simulink model "new"  (R2023a)
settings: Solver=VariableStepAuto  StartTime=0.0  StopTime=4  RelTol=1e-3
values from neighbouring files (symbols this model uses):
  B = 0.0024    [I-PD_pole-placement.mat]    (also in PIV.mat; dobre_pid.mat; exam3.m; exam3_2.m)
  J_m = 0.005    [I-PD_pole-placement.mat]    (also in PIV.mat; dobre_pid.mat; exam3.m; exam3_2.m)
  k_i = 67.5    [I-PD_pole-placement.mat]    (also in PIV.mat = 2.36572; dobre_pid.mat = 0.0660293176822; exam3.m = 4.828; exam3_2.m)
  k_p = 7.6815    [I-PD_pole-placement.mat]    (also in PIV.mat = 5.79950289975; dobre_pid.mat = 8.78704740486; exam3.m = 8.2850041425; exam3_2.m)
  k_v = 0.16658    [PIV.mat]    (also in exam3.m = 0.239)
  M_n = 6.4    [I-PD_pole-placement.mat]    (also in PIV.mat; dobre_pid.mat; exam3.m; exam3_2.m)
  M_z0 = 0.033    [I-PD_pole-placement.mat]    (also in PIV.mat; dobre_pid.mat; exam3.m; exam3_2.m)
  Nel = 10000    [I-PD_pole-placement.mat]    (also in PIV.mat; dobre_pid.mat; exam3.m; exam3_2.m)
  T_n = 0.015    [I-PD_pole-placement.mat]    (also in PIV.mat; dobre_pid.mat; exam3.m; exam3_2.m)
  Tvz = 0.004    [I-PD_pole-placement.mat]    (also in PIV.mat; dobre_pid.mat; exam3.m; exam3_2.m)
undefined symbols (not defined in the file or in its folder): DiscIntNeverNeededParam
settings Model: Creator=laptop  LastModifiedBy=laptop

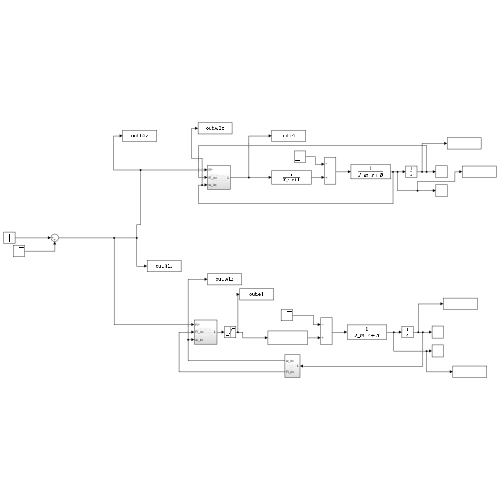
[thumbnail: Simulink's stored preview of the top-level diagram]
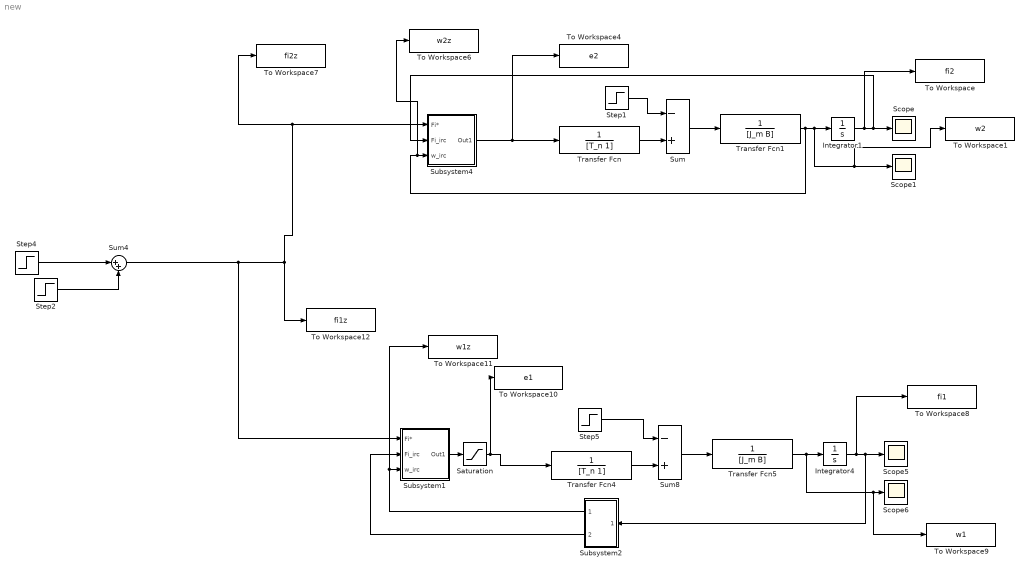
== system new ==
  Integrator1 : Integrator
  Integrator4 : Integrator
  Saturation : Saturate  UpperLimit=M_n*0.75  LowerLimit=-M_n*0.75
  Scope{,1,5..6} (4 alike) : Scope
  Step1 : Step  Time=3  After=M_z0  SampleTime=0
  Step2 : Step  Time=2  After=100  SampleTime=0
  Step4 : Step  After=50  SampleTime=0
  Step5 : Step  Time=3  After=M_z0  SampleTime=0
  Subsystem1 : Subsystem
  Subsystem2 : Subsystem
  Subsystem4 : Subsystem
  Sum : Sum  Inputs=-+
  Sum4 : Sum  Inputs=|++
  Sum8 : Sum  Inputs=-+
  To Workspace : ToWorkspace  VariableName=fi2  SaveFormat=Timeseries  SampleTime=-1
  To Workspace1 : ToWorkspace  VariableName=w2  SaveFormat=Timeseries  SampleTime=-1
  To Workspace10 : ToWorkspace  VariableName=e1  SaveFormat=Timeseries  SampleTime=-1
  To Workspace11 : ToWorkspace  VariableName=w1z  SaveFormat=Timeseries  SampleTime=-1
  To Workspace12 : ToWorkspace  VariableName=fi1z  SaveFormat=Timeseries  SampleTime=-1
  To Workspace4 : ToWorkspace  VariableName=e2  SaveFormat=Timeseries  SampleTime=-1
  To Workspace6 : ToWorkspace  VariableName=w2z  SaveFormat=Timeseries  SampleTime=-1
  To Workspace7 : ToWorkspace  VariableName=fi2z  SaveFormat=Timeseries  SampleTime=-1
  To Workspace8 : ToWorkspace  VariableName=fi1  SaveFormat=Timeseries  SampleTime=-1
  To Workspace9 : ToWorkspace  VariableName=w1  SaveFormat=Timeseries  SampleTime=-1
  Transfer Fcn : TransferFcn  Denominator=[T_n 1]
  Transfer Fcn1 : TransferFcn  Denominator=[J_m B]
  Transfer Fcn4 : TransferFcn  Denominator=[T_n 1]
  Transfer Fcn5 : TransferFcn  Denominator=[J_m B]
  wires:
  Subsystem2/1(w_irc) -> To Workspace11/1, Subsystem1/3(w_irc)
  Transfer Fcn5/1 -> To Workspace9/1, Scope6/1, Integrator4/1
  Integrator1/1 -> To Workspace/1, Subsystem4/2(Fi_irc), Scope/1
  Integrator4/1 -> To Workspace8/1, Subsystem2/1(In1), Scope5/1
  Subsystem2/2(Fi_irc) -> Subsystem1/2(Fi_irc)
  Step1/1 -> Sum/1
  Step2/1 -> Sum4/2
  Step5/1 -> Sum8/1
  Transfer Fcn/1 -> Sum/2
  Transfer Fcn1/1 -> To Workspace6/1, Subsystem4/3(w_irc), To Workspace1/1, Scope1/1, Integrator1/1
  Subsystem1/1(Out1) -> Saturation/1
  Step4/1 -> Sum4/1
  Saturation/1 -> To Workspace10/1, Transfer Fcn4/1
  Sum4/1 -> Subsystem1/1(Fi*), To Workspace7/1, Subsystem4/1(Fi*), To Workspace12/1
  Subsystem4/1(Out1) -> To Workspace4/1, Transfer Fcn/1
  Sum8/1 -> Transfer Fcn5/1
  Sum/1 -> Transfer Fcn1/1
  Transfer Fcn4/1 -> Sum8/2

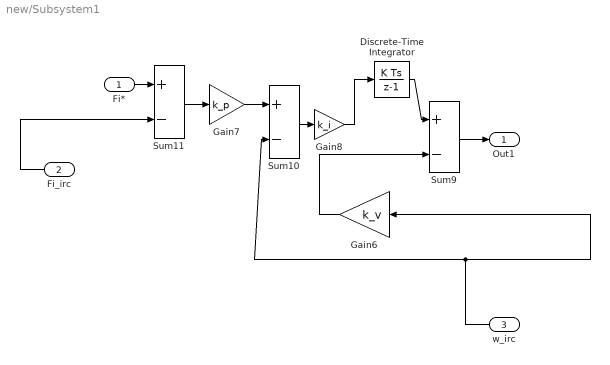
== system new/Subsystem1 ==
  Fi* : Inport
  Fi_irc : Inport  Port=2
  w_irc : Inport  Port=3
  Discrete-Time Integrator : DiscreteIntegrator  SampleTime=Tvz  ICPrevOutput=DiscIntNeverNeededParam  ICPrevScaledInput=DiscIntNeverNeededParam
  Gain6 : Gain  Gain=k_v
  Gain7 : Gain  Gain=k_p
  Gain8 : Gain  Gain=k_i
  Sum10 : Sum  Inputs=+-
  Sum11 : Sum  Inputs=+-
  Sum9 : Sum  Inputs=+-
  Out1 : Outport
  wires:
  Gain6/1 -> Sum9/2
  Sum10/1 -> Gain8/1
  Gain7/1 -> Sum10/1
  Fi_irc/1 -> Sum11/2
  Sum9/1 -> Out1/1
  Gain8/1 -> Discrete-Time Integrator/1
  Discrete-Time Integrator/1 -> Sum9/1
  Sum11/1 -> Gain7/1
  Fi*/1 -> Sum11/1
  w_irc/1 -> Gain6/1, Sum10/2

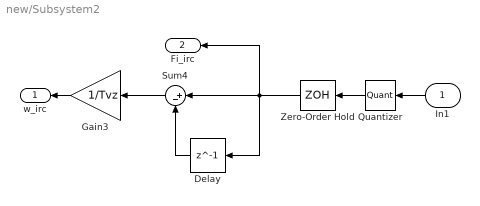
== system new/Subsystem2 ==
  In1 : Inport
  Delay : Delay  DelayLength=1
  Gain3 : Gain  Gain=1/Tvz
  Quantizer : Quantizer  QuantizationInterval=2*pi/Nel
  Sum4 : Sum  Inputs=|+-
  Zero-Order Hold : ZeroOrderHold  SampleTime=Tvz
  w_irc : Outport
  Fi_irc : Outport  Port=2
  wires:
  Sum4/1 -> Gain3/1
  Delay/1 -> Sum4/2
  Zero-Order Hold/1 -> Delay/1, Sum4/1, Fi_irc/1
  In1/1 -> Quantizer/1
  Quantizer/1 -> Zero-Order Hold/1
  Gain3/1 -> w_irc/1

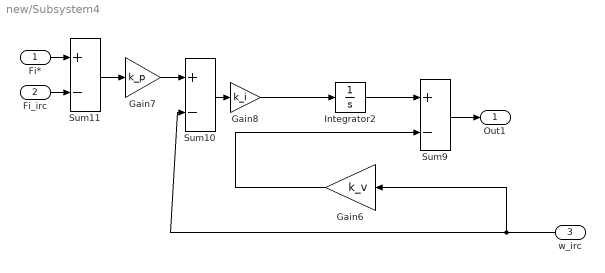
== system new/Subsystem4 ==
  Fi* : Inport
  Fi_irc : Inport  Port=2
  w_irc : Inport  Port=3
  Gain6 : Gain  Gain=k_v
  Gain7 : Gain  Gain=k_p
  Gain8 : Gain  Gain=k_i
  Integrator2 : Integrator
  Sum10 : Sum  Inputs=+-
  Sum11 : Sum  Inputs=+-
  Sum9 : Sum  Inputs=+-
  Out1 : Outport
  wires:
  Gain6/1 -> Sum9/2
  Sum10/1 -> Gain8/1
  Gain7/1 -> Sum10/1
  Fi_irc/1 -> Sum11/2
  Sum9/1 -> Out1/1
  Gain8/1 -> Integrator2/1
  Integrator2/1 -> Sum9/1
  Sum11/1 -> Gain7/1
  Fi*/1 -> Sum11/1
  w_irc/1 -> Sum10/2, Gain6/1
